simulink model "current_model"  (R2023a)
settings: Solver=VariableStepAuto  StartTime=0.0  StopTime=100  RelTol=1e-3
values from neighbouring files (symbols this model uses):
  simulation = 4    [init.m]    (also in plotter.m)
libraries: simulink x3
settings Model: Creator=33769  LastModifiedBy=33769

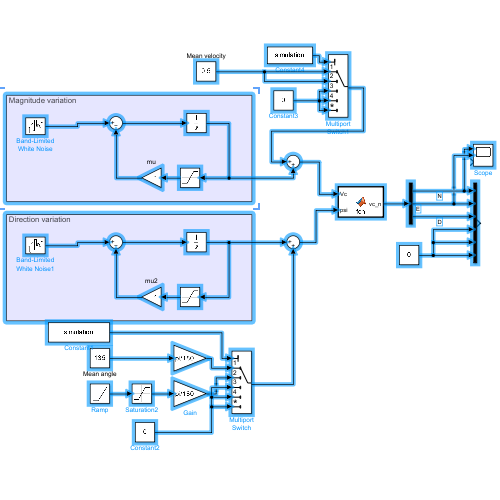
[thumbnail: Simulink's stored preview of the top-level diagram]
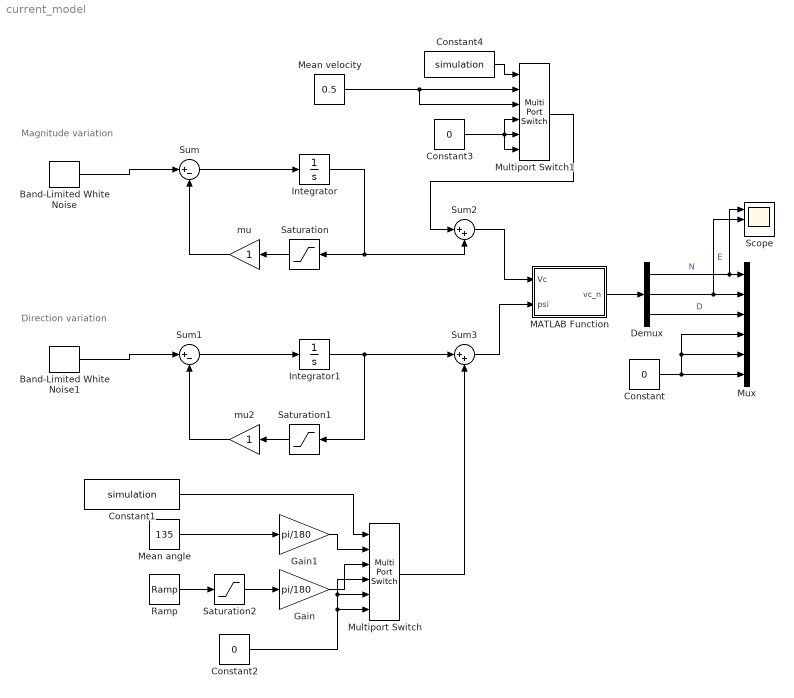
== system current_model ==
  note: Magnitude variation
  note: Direction variation
  Band-Limited White Noise : simulink/Sources/Band-Limited White Noise  Cov=[0]  Ts=0.1  seed=[23341]
  Band-Limited White Noise1 : simulink/Sources/Band-Limited White Noise  Cov=[0]  Ts=0.1  seed=[23341]
  Constant : Constant  Value=0
  Constant1 : Constant  Value=simulation
  Constant2 : Constant  Value=0
  Constant3 : Constant  Value=0
  Constant4 : Constant  Value=simulation
  Demux : Demux  Outputs=3
  Gain : Gain  Gain=pi/180
  Gain1 : Gain  Gain=pi/180
  Integrator : Integrator
  Integrator1 : Integrator
  MATLAB Function : MATLAB Function  TreatAsAtomicUnit=on
  Mean angle : Constant  Value=135
  Mean velocity : Constant  Value=0.5
  Multiport Switch : MultiPortSwitch  Inputs=4  DataPortForDefault=Additional data port  SaturateOnIntegerOverflow=off  InputSameDT=off
  Multiport Switch1 : MultiPortSwitch  Inputs=4  DataPortForDefault=Additional data port  SaturateOnIntegerOverflow=off  InputSameDT=off
  Mux : Mux  Inputs=6
  Ramp : simulink/Sources/Ramp  slope=1  start=0  InitialOutput=0
  Saturation : Saturate  UpperLimit=1  LowerLimit=0
  Saturation1 : Saturate  UpperLimit=pi  LowerLimit=0
  Saturation2 : Saturate  UpperLimit=90  LowerLimit=0
  Scope : Scope  NumInputPorts=3
  Sum : Sum  Inputs=|+-
  Sum1 : Sum  Inputs=|+-
  Sum2 : Sum  Inputs=|++
  Sum3 : Sum  Inputs=|++
  mu : Gain
  mu2 : Gain
  wires:
  Multiport Switch/1 -> Sum3/2
  Gain1/1 -> Multiport Switch/2
  Constant/1 -> Mux/6, Mux/5, Mux/4
  Demux/1 -> Scope/1, Mux/1  "N"
  Demux/3 -> Mux/3  "D"
  Demux/2 -> Scope/2, Mux/2  "E"
  Constant1/1 -> Multiport Switch/1
  mu2/1 -> Sum1/2
  Band-Limited White Noise/1 -> Sum/1
  Integrator1/1 -> Saturation1/1, Sum3/1
  Sum/1 -> Integrator/1
  mu/1 -> Sum/2
  Sum1/1 -> Integrator1/1
  Mean angle/1 -> Gain1/1
  Saturation/1 -> mu/1
  MATLAB Function/1(vc_n) -> Demux/1
  Integrator/1 -> Sum2/2, Saturation/1
  Ramp/1 -> Saturation2/1
  Sum3/1 -> MATLAB Function/2(psi)
  Saturation2/1 -> Gain/1
  Gain/1 -> Multiport Switch/3
  Sum2/1 -> MATLAB Function/1(Vc)
  Saturation1/1 -> mu2/1
  Mean velocity/1 -> Multiport Switch1/3, Multiport Switch1/2
  Band-Limited White Noise1/1 -> Sum1/1
  Constant2/1 -> Multiport Switch/6, Multiport Switch/5, Multiport Switch/4
  Constant3/1 -> Multiport Switch1/4, Multiport Switch1/6, Multiport Switch1/5
  Multiport Switch1/1 -> Sum2/1
  Constant4/1 -> Multiport Switch1/1

== matlab function current_model/MATLAB Function ==
  data: Vc input; vc_n output; psi input
function vc_n = fcn(Vc, psi)


vc_n =[Vc * cos(psi);
     Vc * sin(psi);
     0];
